simulink model "frameTypecast"  (R2024a)
settings: Solver=VariableStepAuto  StartTime=0.0  StopTime=10.0  RelTol=1e-3
libraries: hdlsllib x7, simulink x2
settings Model: Creator=dskap  LastModifiedBy=dskap

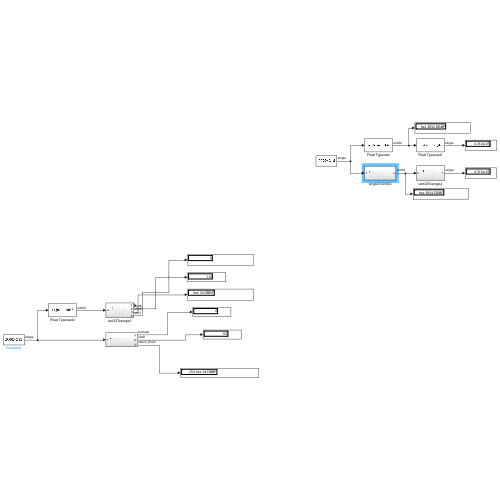
[thumbnail: Simulink's stored preview of the top-level diagram]
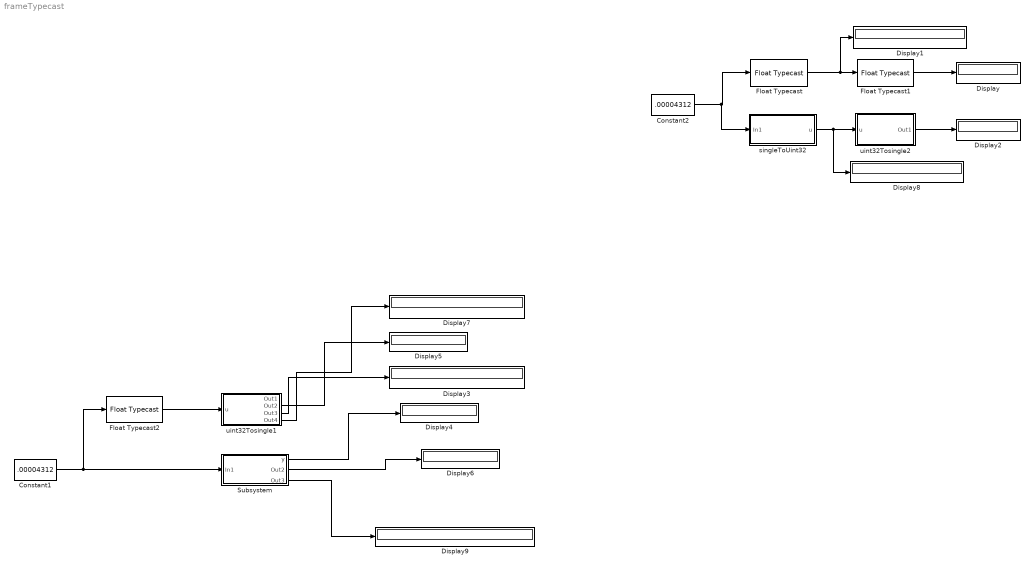
== system frameTypecast ==
  Constant1 : Constant  Value=.00004312  OutDataTypeStr=single
  Constant2 : Constant  Value=.00004312  OutDataTypeStr=single
  Display{,1..9} (10 alike) : Display
      Display1 settings: Format=hex (Stored Integer)
      Display3 settings: Format=hex (Stored Integer)
      Display8 settings: Format=hex (Stored Integer)
      Display9 settings: Format=hex (Stored Integer)
  Float Typecast : FloatTypecast
  Float Typecast1 : FloatTypecast
  Float Typecast2 : FloatTypecast
  Subsystem : Subsystem
  singleToUint32 : Subsystem
  uint32Tosingle1 : Subsystem
  uint32Tosingle2 : Subsystem
  wires:
  Float Typecast/1 -> Display1/1, Float Typecast1/1
  Float Typecast1/1 -> Display/1
  uint32Tosingle2/1(Out1) -> Display2/1
  Constant1/1 -> Subsystem/1(In1), Float Typecast2/1
  uint32Tosingle1/2(Out2) -> Display5/1
  Float Typecast2/1 -> uint32Tosingle1/1(u)
  uint32Tosingle1/3(Out3) -> Display3/1
  uint32Tosingle1/4(Out4) -> Display7/1
  Subsystem/1(y) -> Display4/1
  Subsystem/2(Out2) -> Display6/1
  Subsystem/3(Out3) -> Display9/1
  singleToUint32/1(u) -> Display8/1, uint32Tosingle2/1(u)
  Constant2/1 -> singleToUint32/1(In1), Float Typecast/1

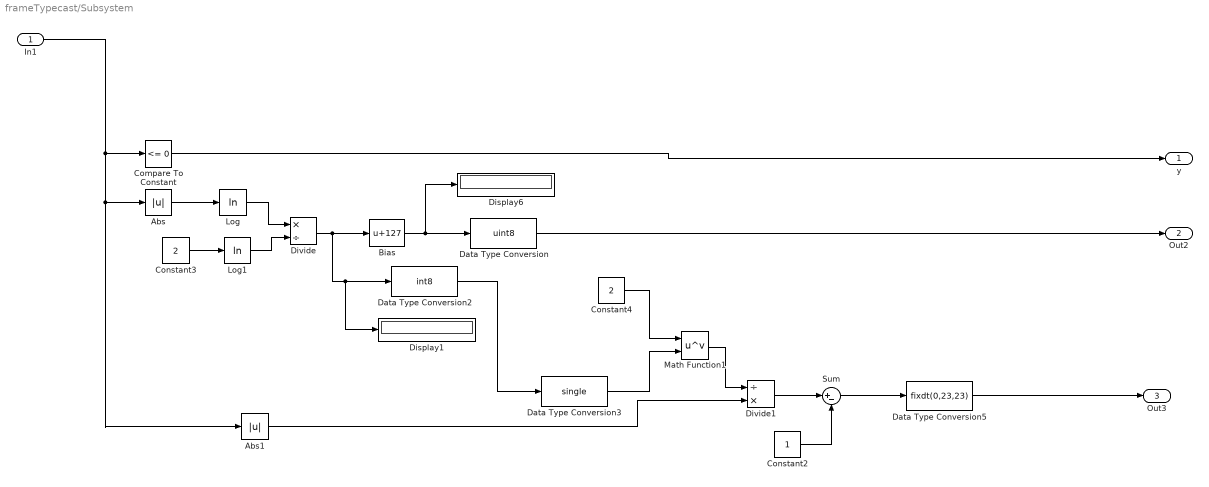
== system frameTypecast/Subsystem ==
  In1 : Inport
  Abs : Abs  SaturateOnIntegerOverflow=off
  Abs1 : Abs  SaturateOnIntegerOverflow=off
  Bias : Bias  Bias=127  SaturateOnIntegerOverflow=off
  Compare To Constant : simulink/Logic and Bit Operations/Compare To Constant  relop=<=  const=0  OutDataTypeStr=boolean
  Constant2 : Constant  OutDataTypeStr=single  SampleTime=-1
  Constant3 : Constant  Value=2  OutDataTypeStr=single  SampleTime=-1
  Constant4 : Constant  Value=2  OutDataTypeStr=single  SampleTime=-1
  Data Type Conversion : DataTypeConversion  OutDataTypeStr=uint8  SaturateOnIntegerOverflow=off  RndMeth=Floor
  Data Type Conversion2 : DataTypeConversion  OutDataTypeStr=int8  SaturateOnIntegerOverflow=off  RndMeth=Floor
  Data Type Conversion3 : DataTypeConversion  OutDataTypeStr=single  SaturateOnIntegerOverflow=off  RndMeth=Floor
  Data Type Conversion5 : DataTypeConversion  OutDataTypeStr=fixdt(0,23,23)  SaturateOnIntegerOverflow=off  RndMeth=Floor
  Display1 : Display
  Display6 : Display
  Divide : Product  Inputs=*/
  Divide1 : Product  Inputs=/*
  Log : Math  Operator=log
  Log1 : Math  Operator=log
  Math Function1 : Math  Operator=pow
  Sum : Sum  Inputs=|+-
  y : Outport
  Out2 : Outport  Port=2
  Out3 : Outport  Port=3
  wires:
  Divide/1 -> Display1/1, Data Type Conversion2/1, Bias/1
  Bias/1 -> Display6/1, Data Type Conversion/1
  Constant3/1 -> Log1/1
  Abs/1 -> Log/1
  Constant4/1 -> Math Function1/1
  Data Type Conversion3/1 -> Math Function1/2
  Math Function1/1 -> Divide1/1
  Log1/1 -> Divide/2
  Log/1 -> Divide/1
  Compare To Constant/1 -> y/1
  In1/1 -> Compare To Constant/1, Abs1/1, Abs/1
  Divide1/1 -> Sum/1
  Sum/1 -> Data Type Conversion5/1
  Data Type Conversion/1 -> Out2/1
  Constant2/1 -> Sum/2
  Abs1/1 -> Divide1/2
  Data Type Conversion2/1 -> Data Type Conversion3/1
  Data Type Conversion5/1 -> Out3/1

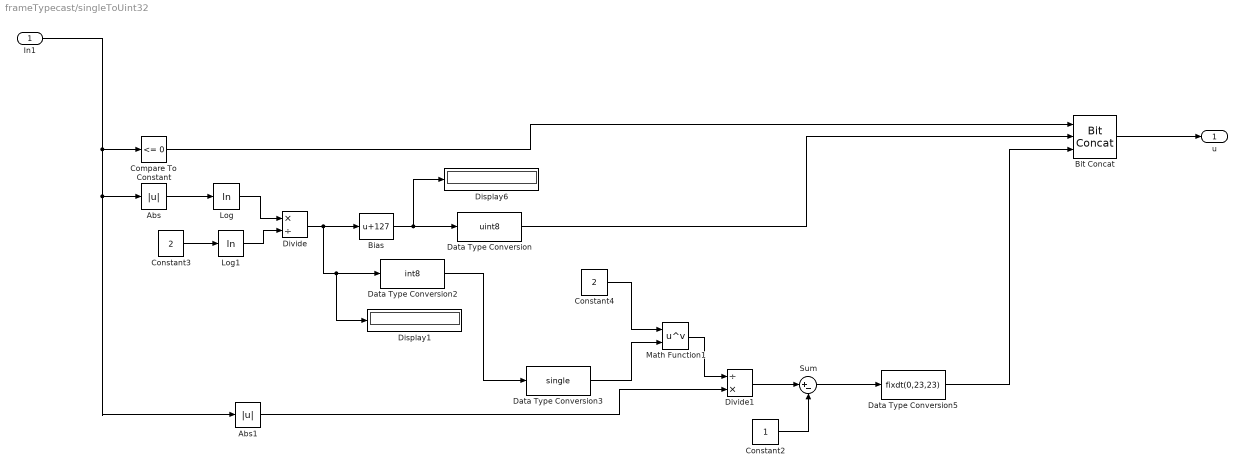
== system frameTypecast/singleToUint32 ==
  In1 : Inport
  Abs : Abs  SaturateOnIntegerOverflow=off
  Abs1 : Abs  SaturateOnIntegerOverflow=off
  Bias : Bias  Bias=127  SaturateOnIntegerOverflow=off
  Bit Concat : hdlsllib/Logic and Bit Operations/Bit Concat  numInputs=3
  Compare To Constant : simulink/Logic and Bit Operations/Compare To Constant  relop=<=  const=0  OutDataTypeStr=boolean
  Constant2 : Constant  OutDataTypeStr=single  SampleTime=-1
  Constant3 : Constant  Value=2  OutDataTypeStr=single  SampleTime=-1
  Constant4 : Constant  Value=2  OutDataTypeStr=single  SampleTime=-1
  Data Type Conversion : DataTypeConversion  OutDataTypeStr=uint8  SaturateOnIntegerOverflow=off  RndMeth=Floor
  Data Type Conversion2 : DataTypeConversion  OutDataTypeStr=int8  SaturateOnIntegerOverflow=off  RndMeth=Floor
  Data Type Conversion3 : DataTypeConversion  OutDataTypeStr=single  SaturateOnIntegerOverflow=off  RndMeth=Floor
  Data Type Conversion5 : DataTypeConversion  OutDataTypeStr=fixdt(0,23,23)  SaturateOnIntegerOverflow=off  RndMeth=Floor
  Display1 : Display
  Display6 : Display
  Divide : Product  Inputs=*/
  Divide1 : Product  Inputs=/*
  Log : Math  Operator=log
  Log1 : Math  Operator=log
  Math Function1 : Math  Operator=pow
  Sum : Sum  Inputs=|+-
  u : Outport
  wires:
  Divide/1 -> Display1/1, Data Type Conversion2/1, Bias/1
  Bias/1 -> Display6/1, Data Type Conversion/1
  Constant3/1 -> Log1/1
  Abs/1 -> Log/1
  Constant4/1 -> Math Function1/1
  Data Type Conversion3/1 -> Math Function1/2
  Math Function1/1 -> Divide1/1
  Log1/1 -> Divide/2
  Log/1 -> Divide/1
  In1/1 -> Compare To Constant/1, Abs1/1, Abs/1
  Divide1/1 -> Sum/1
  Sum/1 -> Data Type Conversion5/1
  Constant2/1 -> Sum/2
  Abs1/1 -> Divide1/2
  Data Type Conversion2/1 -> Data Type Conversion3/1
  Compare To Constant/1 -> Bit Concat/1
  Data Type Conversion/1 -> Bit Concat/2
  Data Type Conversion5/1 -> Bit Concat/3
  Bit Concat/1 -> u/1

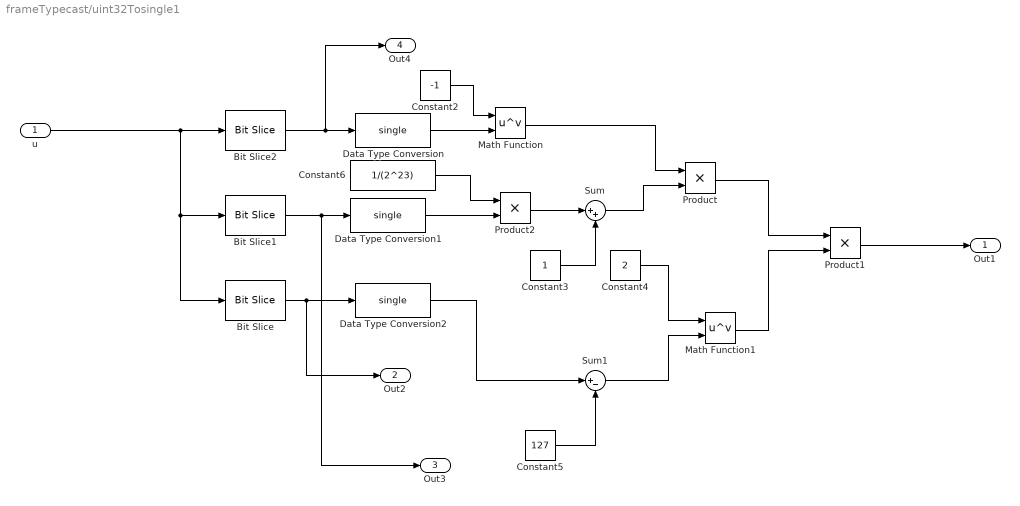
== system frameTypecast/uint32Tosingle1 ==
  u : Inport
  Bit Slice : hdlsllib/Logic and Bit Operations/Bit Slice  lidx=30  ridx=23
  Bit Slice1 : hdlsllib/Logic and Bit Operations/Bit Slice  lidx=22  ridx=0
  Bit Slice2 : hdlsllib/Logic and Bit Operations/Bit Slice  lidx=31  ridx=31
  Constant2 : Constant  Value=-1  OutDataTypeStr=single  SampleTime=-1
  Constant3 : Constant  OutDataTypeStr=single  SampleTime=-1
  Constant4 : Constant  Value=2  OutDataTypeStr=single  SampleTime=-1
  Constant5 : Constant  Value=127  OutDataTypeStr=single  SampleTime=-1
  Constant6 : Constant  Value=1/(2^23)  OutDataTypeStr=single  SampleTime=-1
  Data Type Conversion : DataTypeConversion  OutDataTypeStr=single  SaturateOnIntegerOverflow=off  RndMeth=Floor
  Data Type Conversion1 : DataTypeConversion  OutDataTypeStr=single  SaturateOnIntegerOverflow=off  RndMeth=Floor
  Data Type Conversion2 : DataTypeConversion  OutDataTypeStr=single  SaturateOnIntegerOverflow=off  RndMeth=Floor
  Math Function : Math  Operator=pow
  Math Function1 : Math  Operator=pow
  Product : Product
  Product1 : Product
  Product2 : Product
  Sum : Sum  Inputs=|++
  Sum1 : Sum  Inputs=|+-
  Out1 : Outport
  Out2 : Outport  Port=2
  Out3 : Outport  Port=3
  Out4 : Outport  Port=4
  wires:
  Constant6/1 -> Product2/1
  Data Type Conversion2/1 -> Sum1/1
  Constant3/1 -> Sum/2
  Data Type Conversion1/1 -> Product2/2
  Product/1 -> Product1/1
  Sum/1 -> Product/2
  Constant2/1 -> Math Function/1
  Bit Slice/1 -> Out2/1, Data Type Conversion2/1
  Math Function/1 -> Product/1
  Constant5/1 -> Sum1/2
  Sum1/1 -> Math Function1/2
  Bit Slice2/1 -> Out4/1, Data Type Conversion/1
  Product2/1 -> Sum/1
  Constant4/1 -> Math Function1/1
  u/1 -> Bit Slice2/1, Bit Slice/1, Bit Slice1/1
  Math Function1/1 -> Product1/2
  Data Type Conversion/1 -> Math Function/2
  Bit Slice1/1 -> Out3/1, Data Type Conversion1/1
  Product1/1 -> Out1/1

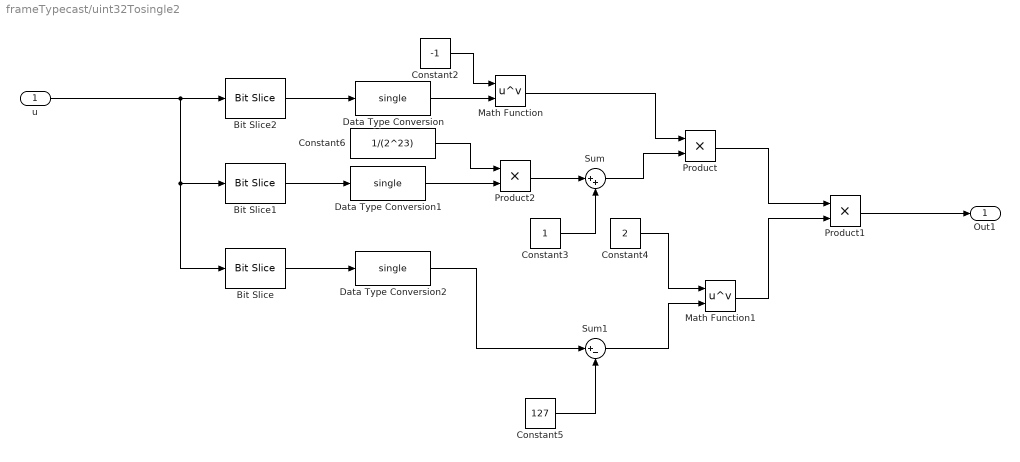
== system frameTypecast/uint32Tosingle2 ==
  u : Inport
  Bit Slice : hdlsllib/Logic and Bit Operations/Bit Slice  lidx=30  ridx=23
  Bit Slice1 : hdlsllib/Logic and Bit Operations/Bit Slice  lidx=22  ridx=0
  Bit Slice2 : hdlsllib/Logic and Bit Operations/Bit Slice  lidx=31  ridx=31
  Constant2 : Constant  Value=-1  OutDataTypeStr=single  SampleTime=-1
  Constant3 : Constant  OutDataTypeStr=single  SampleTime=-1
  Constant4 : Constant  Value=2  OutDataTypeStr=single  SampleTime=-1
  Constant5 : Constant  Value=127  OutDataTypeStr=single  SampleTime=-1
  Constant6 : Constant  Value=1/(2^23)  OutDataTypeStr=single  SampleTime=-1
  Data Type Conversion : DataTypeConversion  OutDataTypeStr=single  SaturateOnIntegerOverflow=off  RndMeth=Floor
  Data Type Conversion1 : DataTypeConversion  OutDataTypeStr=single  SaturateOnIntegerOverflow=off  RndMeth=Floor
  Data Type Conversion2 : DataTypeConversion  OutDataTypeStr=single  SaturateOnIntegerOverflow=off  RndMeth=Floor
  Math Function : Math  Operator=pow
  Math Function1 : Math  Operator=pow
  Product : Product
  Product1 : Product
  Product2 : Product
  Sum : Sum  Inputs=|++
  Sum1 : Sum  Inputs=|+-
  Out1 : Outport
  wires:
  Product1/1 -> Out1/1
  Bit Slice1/1 -> Data Type Conversion1/1
  Data Type Conversion/1 -> Math Function/2
  Math Function1/1 -> Product1/2
  u/1 -> Bit Slice1/1, Bit Slice/1, Bit Slice2/1
  Constant4/1 -> Math Function1/1
  Product2/1 -> Sum/1
  Bit Slice2/1 -> Data Type Conversion/1
  Sum1/1 -> Math Function1/2
  Constant5/1 -> Sum1/2
  Math Function/1 -> Product/1
  Bit Slice/1 -> Data Type Conversion2/1
  Constant2/1 -> Math Function/1
  Sum/1 -> Product/2
  Product/1 -> Product1/1
  Data Type Conversion1/1 -> Product2/2
  Constant3/1 -> Sum/2
  Data Type Conversion2/1 -> Sum1/1
  Constant6/1 -> Product2/1
